simulink model "Properties_Component_Primitives"  (R2012b)
settings: Solver=FixedStepDiscrete  StartTime=0.0  StopTime=10.0  FixedStep=0.1  RelTol=1e-3
libraries: sldvlib x10
settings Model: Creator=Kerianne  LastModifiedBy=Kerianne
settings DataIOCC: SaveFormat=Structure
settings OptimizationCC: InlineParams=on

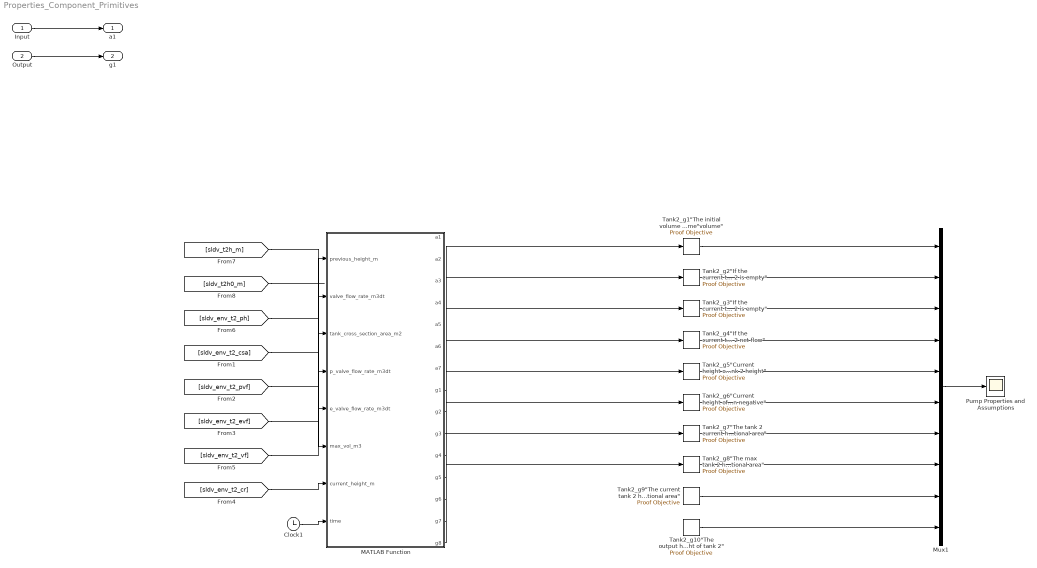
== system Properties_Component_Primitives ==
  Input : Inport  OutDataTypeStr=double
  Output : Inport  Port=2  OutDataTypeStr=double
  Clock1 : Clock
  MATLAB Function : MATLAB Function  TreatAsAtomicUnit=on
  Mux1 : Mux  Inputs=10
  Pump Properties and Assumptions : Scope
      settings: ShowLegends=on
  "Tank2_g1\"The initial volume of tank 2 should be equivalent to the specified initial tank 2 volume\"volume\" " : sldvlib/Objectives and Constraints/Proof Objective  enabled=on  customAVTBlockType=Proof Objective  intervals=true  dispValues=on  outEnabled=on  enableStopSim=off
      settings: AttributesFormatString=%<intervals>
  "Tank2_g10\"The output height of tank 2 should equal the calculated height of tank 2\"" : sldvlib/Objectives and Constraints/Proof Objective  enabled=on  customAVTBlockType=Proof Objective  intervals=true  dispValues=on  outEnabled=on  enableStopSim=off
      settings: AttributesFormatString=%<intervals>
  "Tank2_g2\"If the current tank 2 volume plus the tank 2 net flow is less than the tank 2 minimum volume then tank 2 is empty\" " : sldvlib/Objectives and Constraints/Proof Objective  enabled=on  customAVTBlockType=Proof Objective  intervals=true  dispValues=on  outEnabled=on  enableStopSim=off
      settings: AttributesFormatString=%<intervals>
  "Tank2_g3\"If the current tank 2 volume plus the tank 2 net flow is less than the tank 2 minimum volume then tank 2 is empty\"" : sldvlib/Objectives and Constraints/Proof Objective  enabled=on  customAVTBlockType=Proof Objective  intervals=true  dispValues=on  outEnabled=on  enableStopSim=off
      settings: AttributesFormatString=%<intervals>
  "Tank2_g4\"If the current tank 2 volume plus the tank 2 net flow is greater than empty and less than the tank 2 maximum volume then the tank 2 volume changes by the tank 2 net flow\"" : sldvlib/Objectives and Constraints/Proof Objective  enabled=on  customAVTBlockType=Proof Objective  intervals=true  dispValues=on  outEnabled=on  enableStopSim=off
      settings: AttributesFormatString=%<intervals>
  "Tank2_g5\"Current height of tank 2 is equal or less than the max tank 2 height\"" : sldvlib/Objectives and Constraints/Proof Objective  enabled=on  customAVTBlockType=Proof Objective  intervals=true  dispValues=on  outEnabled=on  enableStopSim=off
      settings: AttributesFormatString=%<intervals>
  "Tank2_g6\"Current height of tank 2 is non negative\"" : sldvlib/Objectives and Constraints/Proof Objective  enabled=on  customAVTBlockType=Proof Objective  intervals=true  dispValues=on  outEnabled=on  enableStopSim=off
      settings: AttributesFormatString=%<intervals>
  "Tank2_g7\"The tank 2 current height is equal to the tank 2 current volume divided by the tank 2 cross sectional area\" " : sldvlib/Objectives and Constraints/Proof Objective  enabled=on  customAVTBlockType=Proof Objective  intervals=true  dispValues=on  outEnabled=on  enableStopSim=off
      settings: AttributesFormatString=%<intervals>
  "Tank2_g8\"The max tank 2 height is equal to the max tank 2 volume divided by tank 2 cross sectional area\"" : sldvlib/Objectives and Constraints/Proof Objective  enabled=on  customAVTBlockType=Proof Objective  intervals=true  dispValues=on  outEnabled=on  enableStopSim=off
      settings: AttributesFormatString=%<intervals>
  "Tank2_g9\"The current tank 2 height is the current tank 2 volume divided by the tank 2 cross sectional area\"" : sldvlib/Objectives and Constraints/Proof Objective  enabled=on  customAVTBlockType=Proof Objective  intervals=true  dispValues=on  outEnabled=on  enableStopSim=off
      settings: AttributesFormatString=%<intervals>
  a1 : Outport  OutDataTypeStr=boolean
  g1 : Outport  Port=2  OutDataTypeStr=boolean
  wires:
  Input/1 -> a1/1
  Output/1 -> g1/1
  "Tank2_g9\"The current tank 2 height is the current tank 2 volume divided by the tank 2 cross sectional area\""/1 -> Mux1/9
  MATLAB Function/10(g3) -> "Tank2_g3\"If the current tank 2 volume plus the tank 2 net flow is less than the tank 2 minimum volume then tank 2 is empty\""/1
  MATLAB Function/8(g1) -> "Tank2_g1\"The initial volume of tank 2 should be equivalent to the specified initial tank 2 volume\"volume\" "/1
  Clock1/1 -> MATLAB Function/8(time)
  MATLAB Function/11(g4) -> "Tank2_g4\"If the current tank 2 volume plus the tank 2 net flow is greater than empty and less than the tank 2 maximum volume then the tank 2 volume changes by the tank 2 net flow\""/1
  "Tank2_g1\"The initial volume of tank 2 should be equivalent to the specified initial tank 2 volume\"volume\" "/1 -> Mux1/1
  MATLAB Function/12(g5) -> "Tank2_g5\"Current height of tank 2 is equal or less than the max tank 2 height\""/1
  MATLAB Function/13(g6) -> "Tank2_g6\"Current height of tank 2 is non negative\""/1
  MATLAB Function/14(g7) -> "Tank2_g7\"The tank 2 current height is equal to the tank 2 current volume divided by the tank 2 cross sectional area\" "/1
  Mux1/1 -> Pump Properties and Assumptions/1
  MATLAB Function/9(g2) -> "Tank2_g2\"If the current tank 2 volume plus the tank 2 net flow is less than the tank 2 minimum volume then tank 2 is empty\" "/1
  MATLAB Function/15(g8) -> "Tank2_g8\"The max tank 2 height is equal to the max tank 2 volume divided by tank 2 cross sectional area\""/1
  ? -> "Tank2_g9\"The current tank 2 height is the current tank 2 volume divided by the tank 2 cross sectional area\""/1
  ? -> "Tank2_g10\"The output height of tank 2 should equal the calculated height of tank 2\""/1
  "Tank2_g2\"If the current tank 2 volume plus the tank 2 net flow is less than the tank 2 minimum volume then tank 2 is empty\" "/1 -> Mux1/2
  "Tank2_g3\"If the current tank 2 volume plus the tank 2 net flow is less than the tank 2 minimum volume then tank 2 is empty\""/1 -> Mux1/3
  "Tank2_g4\"If the current tank 2 volume plus the tank 2 net flow is greater than empty and less than the tank 2 maximum volume then the tank 2 volume changes by the tank 2 net flow\""/1 -> Mux1/4
  "Tank2_g5\"Current height of tank 2 is equal or less than the max tank 2 height\""/1 -> Mux1/5
  "Tank2_g6\"Current height of tank 2 is non negative\""/1 -> Mux1/6
  "Tank2_g7\"The tank 2 current height is equal to the tank 2 current volume divided by the tank 2 cross sectional area\" "/1 -> Mux1/7
  "Tank2_g8\"The max tank 2 height is equal to the max tank 2 volume divided by tank 2 cross sectional area\""/1 -> Mux1/8
  "Tank2_g10\"The output height of tank 2 should equal the calculated height of tank 2\""/1 -> Mux1/10
  [sldv_env_t2_ph] -> MATLAB Function/1(previous_height_m)
  [sldv_env_t2_csa] -> MATLAB Function/3(tank_cross_section_area_m2)
  [sldv_env_t2_pvf] -> MATLAB Function/4(p_valve_flow_rate_m3dt)
  [sldv_env_t2_evf] -> MATLAB Function/5(e_valve_flow_rate_m3dt)
  [sldv_env_t2_vf] -> MATLAB Function/2(valve_flow_rate_m3dt)
  [sldv_env_t2_cr] -> MATLAB Function/7(current_height_m)
  [sldv_t2h_m] -> MATLAB Function/6(max_vol_m3)
  [sldv_t2h0_m] -> ?

== matlab function Properties_Component_Primitives/MATLAB Function ==
  data: a1 output; a2 output; a3 output; a4 output; a5 output; a6 output; a7 output; previous_height_m input; valve_flow_rate_m3dt input; tank_cross_section_area_m2 input; p_valve_flow_rate_m3dt input; e_valve_flow_rate_m3dt input; max_vol_m3 input; g1 output; current_height_m input; time input; g2 output; g3 output; g4 output; g5 output; g6 output; g7 output; g8 output
function [a1, a2, a3, a4, a5, a6, a7, g1, g2, g3, g4, g5, g6, g7, g8]   = verification_condition(previous_height_m, valve_flow_rate_m3dt, tank_cross_section_area_m2, p_valve_flow_rate_m3dt, e_valve_flow_rate_m3dt, max_vol_m3, current_height_m, time)

% Updated 27 Feb 2015 from 20150205 tank2.aadl

persistent pre_max_vol_m3
if isempty(pre_max_vol_m3)
    pre_max_vol_m3 = max_vol_m3;
end
persistent pre_tank_cross_section_area_m2
if isempty(pre_tank_cross_section_area_m2)
    pre_tank_cross_section_area_m2 = tank_cross_section_area_m2;
end

tank_height_m = max_vol_m3/tank_cross_section_area_m2;
current_volume_m3 = current_height_m*tank_cross_section_area_m2;
previous_volume_m3 = previous_height_m*tank_cross_section_area_m2;
net_flow_m3dt = valve_flow_rate_m3dt-p_valve_flow_rate_m3dt-e_valve_flow_rate_m3dt;
initial_height_m = 0.0;

% Assumptions
% assume "Valve flow rate is positive"
a1 = valve_flow_rate_m3dt >= 0.0;
% assume "Tank cross section area is positive"
a2 = tank_cross_section_area_m2 >= 0.0;
% assume "Tank cross section area is constant"
a3 = pre_tank_cross_section_area_m2 == tank_cross_section_area_m2;
% assume "P valve flow rate is positive"
a4 = p_valve_flow_rate_m3dt >= 0.0;
% assume "E valve flow rate is positive"
a5 = e_valve_flow_rate_m3dt >= 0.0;
% assume "Tank volume is positive"
a6 = max_vol_m3 >= 0;
% assume "Tank volume is constant"
a7 = pre_max_vol_m3 == max_vol_m3;
% previous hight - taken out


			
% guarantee "The initial volume of tank 2 should be equivalent to the specified initial tank 2 volume"
g1 = initially_empty(initial_height_m, previous_height_m,time,tank_cross_section_area_m2);
% guarantee "If the current tank 2 volume plus the tank 2 net flow is greater than the tank 2 maximum volume then tank 2 is full"
g2 = full_cond(current_volume_m3, net_flow_m3dt, max_vol_m3);	
% guarantee "If the current tank 2 volume plus the tank 2 net flow is less than the tank 2 minimum volume then tank 2 is empty" 
g3 = empty_cond(current_volume_m3, net_flow_m3dt);
% guarantee "If the current tank 2 volume plus the tank 2 net flow is greater than empty and less than the tank 2 maximum volume then the tank 2 volume changes by the tank 2 net flow"
g4 = tank_volume_update(current_volume_m3, net_flow_m3dt, max_vol_m3, previous_volume_m3);
% guarantee "Current height of tank 2 is equal or less than the max tank 2 height" 
g5 = tank_less_or_equal_full(current_height_m, tank_height_m);
% guarantee "Current height of tank 2 is non negative"
g6 = current_height_m >= 0.0;
% guarantee "The tank 2 current height is equal to the tank 2 current volume divided by the tank 2 cross sectional area" 
g7 = math_check(current_height_m, current_volume_m3, tank_cross_section_area_m2);
% guarantee "The max tank 2 height is equal to the max tank 2 volume divided by tank 2 cross sectional area"
g8 = math_check_2(tank_height_m, max_vol_m3, tank_cross_section_area_m2); 
% % guarantee "The current tank 2 height is the current tank 2 volume divided by the tank 2 cross sectional area"
% g9 = math_check_3(current_height_m, current_volume_m3, tank_cross_section_area_m2);
% % guarantee "The output height of tank 2 should equal the calculated height of tank 2"
% g10 = math_check_4(current_height_m, p_valve_flow_rate_m3dt, e_valve_flow_rate_m3dt, valve_flow_rate_m3dt, tank_cross_section_area_m2, previous_height_m);

function c = implies(a,b)      
     c = ((not (a)) || b);
% g1 "The initial volume of tank 2 should be equivalent to the specified initial tank 2 volume"
function result = initially_empty(initial_height_m, previous_height_m, time, tank_cross_section_area_m2)
    UnderThisCondition = (time == 0.0);
    ResultShouldBe = (previous_height_m*tank_cross_section_area_m2 == initial_height_m*tank_cross_section_area_m2);
    result = implies(UnderThisCondition, ResultShouldBe);
% g2 "If the current tank 2 volume plus the tank 2 net flow is greater than the tank 2 maximum volume then tank 2 is full"
function result = full_cond(current_volume_m3, net_flow_m3dt, tank_volume_m3)
    UnderThisCondition = (current_volume_m3 + net_flow_m3dt >= tank_volume_m3);
    ResultShouldBe = (current_volume_m3 == tank_volume_m3);
    result = implies(UnderThisCondition, ResultShouldBe);
% g3 "If the current tank 2 volume plus the tank 2 net flow is less than the tank 2 minimum volume then tank 2 is empty" 
function result = empty_cond(current_volume_m3, net_flow_m3dt)    
    UnderThisCondition = (current_volume_m3 + net_flow_m3dt <= 0.0);
    ResultShouldBe = (current_volume_m3 == 0.0);
    result = implies(UnderThisCondition, ResultShouldBe);
% g4 "If the current tank 2 volume plus the tank 2 net flow is greater than empty and less than the tank 2 maximum volume then the tank 2 volume changes by the tank 2 net flow"
function result = tank_volume_update(current_volume_m3, net_flow_m3dt, tank_volume_m3, previous_volume_m3)   
    UnderThisCondition = ((current_volume_m3 + net_flow_m3dt <= tank_volume_m3) && (current_volume_m3 + net_flow_m3dt >= 0.0));
    ResultShouldBe = (current_volume_m3 == previous_volume_m3 + net_flow_m3dt);
    result = implies(UnderThisCondition, ResultShouldBe);
% g5 "Current height of tank 2 is equal or less than the max tank 2 height"
function result = tank_less_or_equal_full(current_height_m, tank_height_m)   
    result = (current_height_m <= tank_height_m);
% g6 "Current height of tank 2 is non negative"
function result = tank_height_not_negative(current_height_m)   
    result = (current_height_m >= 0);
% g7 "The tank 2 current height is equal to the tank 2 current volume divided by the tank 2 cross sectional area" 
function result =  math_check(current_height_m, current_volume_m3, tank_cross_section_area_m2)
    result = (current_height_m == current_volume_m3 / tank_cross_section_area_m2);
% g8 "The max tank 2 height is equal to the max tank 2 volume divided by tank 2 cross sectional area"
function result =  math_check_2(tank_height_m, tank_volume_m3, tank_cross_section_area_m2)
    result = (tank_height_m == tank_volume_m3/ tank_cross_section_area_m2);
% g9 "The current tank 2 height is the current tank 2 volume divided by the tank 2 cross sectional area"
function result = math_check_3(current_height_m, current_volume_m3, tank_cross_section_area_m2)
 	result = (current_height_m == current_volume_m3 / tank_cross_section_area_m2);
% g10 "The output height of tank 2 should equal the calculated height of tank 2"
function result = math_check_4(current_height_m, p_valve_flow_rate_m3dt, e_valve_flow_rate_m3dt, valve_flow_rate_m3dt, tank_cross_section_area_m2, previous_height_m)
    result = (current_height_m == ((valve_flow_rate_m3dt-p_valve_flow_rate_m3dt-e_valve_flow_rate_m3dt)/tank_cross_section_area_m2) +previous_height_m);
